simulink model "car_kine1"  (R2019a)
settings: Solver=VariableStepAuto  StartTime=0.0  StopTime=20.0  RelTol=1e-3
libraries: simulink x1
settings Model: Creator=mi  LastModifiedBy=mi

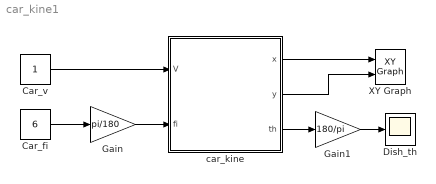
== system car_kine1 ==
  Car_fi : Constant  Value=6
  Car_v : Constant
  "Dish_th " : Scope
  Gain : Gain  Gain=pi/180
  Gain1 : Gain  Gain=180/pi
  XY Graph : simulink/Sinks/XY Graph  xmin=-3  xmax=3  ymin=-0.2  ymax=5.2  st=-1
  car_kine : Subsystem  mask{L=0.254}
      mask prompts: L "小车车长L(米)"
  wires:
  car_kine/3("th ") -> Gain1/1
  Gain1/1 -> "Dish_th "/1
  Car_v/1 -> car_kine/1(V)
  Gain/1 -> car_kine/2(fi)
  car_kine/1(x) -> XY Graph/1
  car_kine/2(y) -> XY Graph/2
  Car_fi/1 -> Gain/1

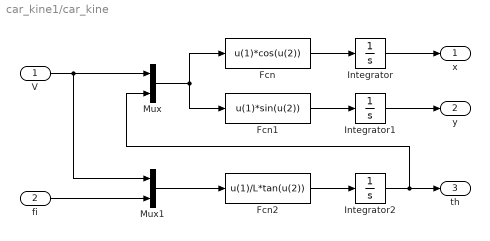
== system car_kine1/car_kine ==
  V : Inport
  fi : Inport  Port=2
  Fcn : Fcn  Expr=u(1)*cos(u(2))
  Fcn1 : Fcn  Expr=u(1)*sin(u(2))
  Fcn2 : Fcn  Expr=u(1)/L*tan(u(2))
  Integrator : Integrator
  Integrator1 : Integrator
  Integrator2 : Integrator
  Mux : Mux  Inputs=2
  Mux1 : Mux  Inputs=2
  x : Outport
  y : Outport  Port=2
  "th " : Outport  Port=3
  wires:
  Integrator2/1 -> "th "/1, Mux/2
  Fcn/1 -> Integrator/1
  Mux1/1 -> Fcn2/1
  Fcn2/1 -> Integrator2/1
  fi/1 -> Mux1/2
  Integrator1/1 -> y/1
  Mux/1 -> Fcn/1, Fcn1/1
  V/1 -> Mux1/1, Mux/1
  Integrator/1 -> x/1
  Fcn1/1 -> Integrator1/1
